simulink library "environmentManta4Rot_cl"  (R2020a)
settings: Solver=VariableStepAuto  StartTime=0.0  StopTime=10.0  RelTol=1e-3
undefined symbols (not defined in the file or in its folder): initializeBussesFromBlock
libraries: flowcalculation_cl x4
settings Model: Creator=mcobb  LastModifiedBy=John Jr
settings DataIOCC: ReturnWorkspaceOutputs=off
settings DebuggingCC: ArithmeticOperatorsInVariantConditions=warning
settings SFSimCC: CustomCodeUndefinedFunction=UseInterfaceOnly

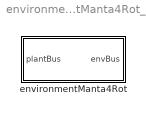
== system environmentManta4Rot_cl ==
  environmentManta4Rot : Subsystem  LoadFcn=initializeBussesFromBlock(gcb)  InitFcn=initializeBussesFromBlock(gcb)  StartFcn=initializeBussesFromBlock(gcb)
      settings: MinAlgLoopOccurrences=on

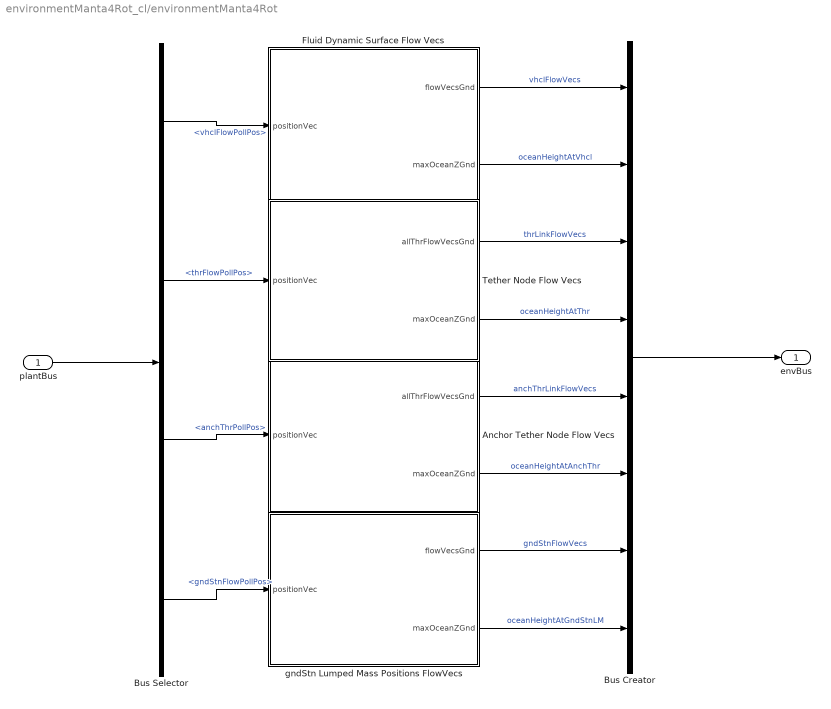
== system environmentManta4Rot_cl/environmentManta4Rot ==
  plantBus : Inport  OutDataTypeStr=Bus: plantBus
  Anchor Tether Node Flow Vecs : Subsystem
  Bus Creator : BusCreator  Inputs=8  OutDataTypeStr=Bus: envBus  NonVirtualBus=on
  Bus Selector : BusSelector  OutputSignals=vhclFlowPollPos,thrFlowPollPos,anchThrPollPos,gndStnFlowPollPos
  Fluid Dynamic Surface Flow Vecs : Subsystem
      settings: MinAlgLoopOccurrences=on
  Tether Node Flow Vecs : Subsystem
      settings: MinAlgLoopOccurrences=on
  gndStn Lumped Mass Positions FlowVecs : Subsystem
      settings: MinAlgLoopOccurrences=on
  envBus : Outport  OutDataTypeStr=Bus: envBus  VectorParamsAs1DForOutWhenUnconnected=off
  wires:
  Bus Selector/1 -> Fluid Dynamic Surface Flow Vecs/1(positionVec)  "<vhclFlowPollPos>"
  Fluid Dynamic Surface Flow Vecs/1(flowVecsGnd) -> Bus Creator/1  "vhclFlowVecs"
  Bus Creator/1 -> envBus/1
  Bus Selector/3 -> Anchor Tether Node Flow Vecs/1(positionVec)  "<anchThrPollPos>"
  Bus Selector/2 -> Tether Node Flow Vecs/1(positionVec)  "<thrFlowPollPos>"
  plantBus/1 -> Bus Selector/1
  Bus Selector/4 -> gndStn Lumped Mass Positions FlowVecs/1(positionVec)  "<gndStnFlowPollPos>"
  gndStn Lumped Mass Positions FlowVecs/2(maxOceanZGnd) -> Bus Creator/8  "oceanHeightAtGndStnLM"
  Tether Node Flow Vecs/1(allThrFlowVecsGnd) -> Bus Creator/3  "thrLinkFlowVecs"
  Anchor Tether Node Flow Vecs/1(allThrFlowVecsGnd) -> Bus Creator/5  "anchThrLinkFlowVecs"
  gndStn Lumped Mass Positions FlowVecs/1(flowVecsGnd) -> Bus Creator/7  "gndStnFlowVecs"
  Anchor Tether Node Flow Vecs/2(maxOceanZGnd) -> Bus Creator/6  "oceanHeightAtAnchThr"
  Tether Node Flow Vecs/2(maxOceanZGnd) -> Bus Creator/4  "oceanHeightAtThr"
  Fluid Dynamic Surface Flow Vecs/2(maxOceanZGnd) -> Bus Creator/2  "oceanHeightAtVhcl"

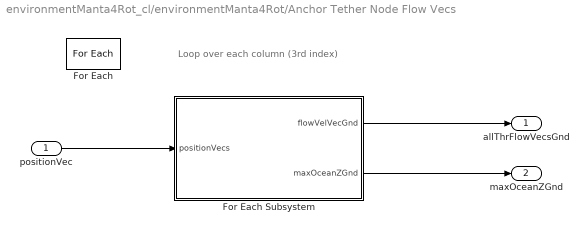
== system environmentManta4Rot_cl/environmentManta4Rot/Anchor Tether Node Flow Vecs ==
  note: Loop over each column (3rd index)
  positionVec : Inport  Partition=on  PartitionDimension=3  PartitionWidth=1  PartitionOffset=0
  For Each : ForEach  DisableCoverage=on
  For Each Subsystem : Subsystem
      settings: MinAlgLoopOccurrences=on
  allThrFlowVecsGnd : Outport  ConcatenationDimension=3  VectorParamsAs1DForOutWhenUnconnected=off
  maxOceanZGnd : Outport  Port=2  ConcatenationDimension=1  VectorParamsAs1DForOutWhenUnconnected=off
  wires:
  positionVec/1 -> For Each Subsystem/1(positionVecs)
  For Each Subsystem/1(flowVelVecGnd) -> allThrFlowVecsGnd/1
  For Each Subsystem/2(maxOceanZGnd) -> maxOceanZGnd/1

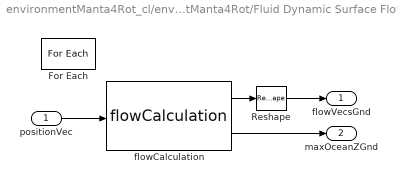
== system environmentManta4Rot_cl/environmentManta4Rot/Fluid Dynamic Surface Flow Vecs ==
  positionVec : Inport  Partition=on  PartitionDimension=2  PartitionWidth=1  PartitionOffset=0
  For Each : ForEach  DisableCoverage=on
  Reshape : Reshape  OutputDimensionality=Column vector (2-D)
  flowCalculation : flowcalculation_cl/flowCalculation  SystemSampleTime=-1
  flowVecsGnd : Outport  ConcatenationDimension=2  VectorParamsAs1DForOutWhenUnconnected=off
  maxOceanZGnd : Outport  Port=2  ConcatenationDimension=1  VectorParamsAs1DForOutWhenUnconnected=off
  wires:
  positionVec/1 -> flowCalculation/1
  flowCalculation/1 -> Reshape/1
  Reshape/1 -> flowVecsGnd/1
  flowCalculation/2 -> maxOceanZGnd/1

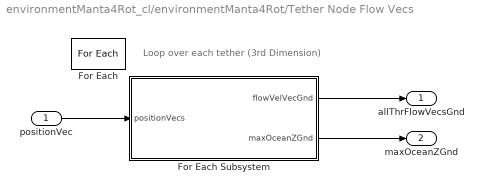
== system environmentManta4Rot_cl/environmentManta4Rot/Tether Node Flow Vecs ==
  note: Loop over each tether (3rd Dimension)
  positionVec : Inport  Partition=on  PartitionDimension=3  PartitionWidth=1  PartitionOffset=0
  For Each : ForEach  DisableCoverage=on
  For Each Subsystem : Subsystem
      settings: MinAlgLoopOccurrences=on
  allThrFlowVecsGnd : Outport  ConcatenationDimension=3  VectorParamsAs1DForOutWhenUnconnected=off
  maxOceanZGnd : Outport  Port=2  ConcatenationDimension=1  VectorParamsAs1DForOutWhenUnconnected=off
  wires:
  For Each Subsystem/1(flowVelVecGnd) -> allThrFlowVecsGnd/1
  positionVec/1 -> For Each Subsystem/1(positionVecs)
  For Each Subsystem/2(maxOceanZGnd) -> maxOceanZGnd/1

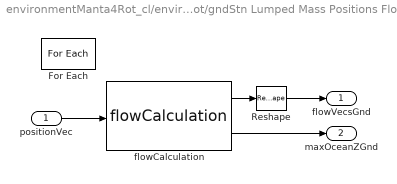
== system environmentManta4Rot_cl/environmentManta4Rot/gndStn Lumped Mass Positions FlowVecs ==
  positionVec : Inport  Partition=on  PartitionDimension=2  PartitionWidth=1  PartitionOffset=0
  For Each : ForEach  DisableCoverage=on
  Reshape : Reshape  OutputDimensionality=Column vector (2-D)
  flowCalculation : flowcalculation_cl/flowCalculation  SystemSampleTime=-1  Latency=0  AutoFrameSizeCalculation=off
  flowVecsGnd : Outport  ConcatenationDimension=2  VectorParamsAs1DForOutWhenUnconnected=off
  maxOceanZGnd : Outport  Port=2  ConcatenationDimension=1  VectorParamsAs1DForOutWhenUnconnected=off
  wires:
  flowCalculation/2 -> maxOceanZGnd/1
  Reshape/1 -> flowVecsGnd/1
  flowCalculation/1 -> Reshape/1
  positionVec/1 -> flowCalculation/1

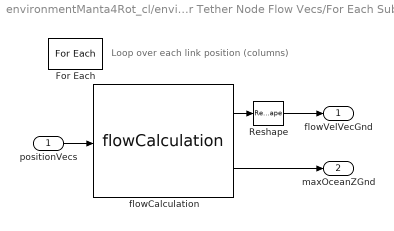
== system environmentManta4Rot_cl/environmentManta4Rot/Anchor Tether Node Flow Vecs/For Each Subsystem ==
  note: Loop over each link position (columns)
  positionVecs : Inport  Partition=on  PartitionDimension=2  PartitionWidth=1  PartitionOffset=0
  For Each : ForEach  DisableCoverage=on
  Reshape : Reshape  OutputDimensionality=Column vector (2-D)
  flowCalculation : flowcalculation_cl/flowCalculation  SystemSampleTime=-1  Latency=0  AutoFrameSizeCalculation=off
  flowVelVecGnd : Outport  ConcatenationDimension=2  VectorParamsAs1DForOutWhenUnconnected=off
  maxOceanZGnd : Outport  Port=2  ConcatenationDimension=1  VectorParamsAs1DForOutWhenUnconnected=off
  wires:
  flowCalculation/1 -> Reshape/1
  Reshape/1 -> flowVelVecGnd/1
  positionVecs/1 -> flowCalculation/1
  flowCalculation/2 -> maxOceanZGnd/1

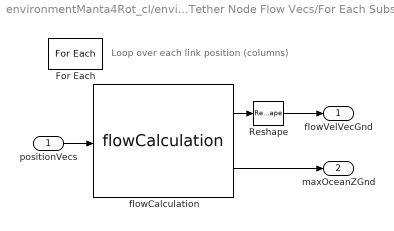
== system environmentManta4Rot_cl/environmentManta4Rot/Tether Node Flow Vecs/For Each Subsystem ==
  note: Loop over each link position (columns)
  positionVecs : Inport  Partition=on  PartitionDimension=2  PartitionWidth=1  PartitionOffset=0
  For Each : ForEach  DisableCoverage=on
  Reshape : Reshape  OutputDimensionality=Column vector (2-D)
  flowCalculation : flowcalculation_cl/flowCalculation  SystemSampleTime=-1
  flowVelVecGnd : Outport  ConcatenationDimension=2  VectorParamsAs1DForOutWhenUnconnected=off
  maxOceanZGnd : Outport  Port=2  ConcatenationDimension=1  VectorParamsAs1DForOutWhenUnconnected=off
  wires:
  flowCalculation/1 -> Reshape/1
  Reshape/1 -> flowVelVecGnd/1
  positionVecs/1 -> flowCalculation/1
  flowCalculation/2 -> maxOceanZGnd/1
